simulink model "BL_CollectivePitch_Shutdown"  (R2018a)
settings: Solver=FixedStepAuto  StartTime=0.0  StopTime=FA.TMax  RelTol=1e-3
values from neighbouring files (symbols this model uses):
  FaultDelay = 1    [B_DLC_1_1.m]    (also in B_DLC_1_3.m; B_DLC_1_4.m; B_DLC_1_5.m; B_DLC_2_2.m)
  GenTorqueStopRate = 800/1e3    (= 0.8)    [B_DLC_1_1.m]    (also in B_DLC_1_3.m; B_DLC_1_4.m; B_DLC_1_5.m; B_DLC_2_2.m)
  PitchFaultTime = FA.TMax + 100    [B_DLC_1_1.m]    (also in B_DLC_1_3.m; B_DLC_1_4.m; B_DLC_1_5.m; B_DLC_2_2.m = PitchFaultTimeArray(iFaultTime))
  PitchRampRate1 = 12    [B_DLC_1_1.m]    (also in B_DLC_1_3.m; B_DLC_1_4.m; B_DLC_1_5.m; B_DLC_2_2.m)
  PitchRampRate2 = 2    [B_DLC_1_1.m]    (also in B_DLC_1_3.m; B_DLC_1_4.m; B_DLC_1_5.m; B_DLC_2_2.m)
  PitchRunawayRate = 18    [B_DLC_1_1.m]    (also in B_DLC_1_3.m; B_DLC_1_4.m; B_DLC_1_5.m; B_DLC_2_2.m)
  runawayBlade = 0    [B_DLC_1_1.m]    (also in B_DLC_1_3.m; B_DLC_1_4.m; B_DLC_1_5.m; B_DLC_2_2.m)
  stuckBlade = 0    [B_DLC_1_1.m]    (also in B_DLC_1_3.m; B_DLC_1_4.m; B_DLC_1_5.m; B_DLC_2_2.m)
  YawPzn = Yaw(iYaw)*pi/180    [B_DLC_6_1.m]
  YawRate = 0    [B_DLC_6_1.m]
undefined symbols (not defined in the file or in its folder): Control, DiscIntNeverNeededParam, OLControlParams, OutList, Parameters, PitchControlParams, rpm2radps, S_ConstTq, S_LowBPLim, strmatch, TorqueControlParams
libraries: simulink_extras x1
settings Model: ExtModeTrigMode=oneshot  ExtModeArmWhenConnect=off  Creator=Hazim Namik  LastModifiedBy=dmartin
settings DataIOCC: LimitDataPoints=on  SaveFormat=Array  SignalLoggingName=sigsOut
settings OptimizationCC: BlockReduction=off  BooleanDataType=off  LifeSpan=inf
settings DebuggingCC: SaveWithParameterizedLinksMsg=none  UnderspecifiedInitializationDetection=Classic  MergeDetectMultiDrivingBlocksExec=none  SignalResolutionControl=TryResolveAllWithWarning  AllowSymbolicDim=off  SFUnexpectedBacktrackingDiag=warning  SFNoUnconditionalDefaultTransitionDiag=warning  SFExecutionAtInitializationDiag=none
settings HardwareCC: ProdBitPerPointer=32  ProdBitPerSizeT=32  ProdBitPerPtrDiffT=32  ProdLargestAtomicFloat=None  ProdIntDivRoundTo=Undefined  ProdEndianess=Unspecified  ProdWordSize=32  ProdHWDeviceType=32-bit Generic  TargetBitPerPointer=64  TargetBitPerSizeT=64  TargetBitPerPtrDiffT=64  TargetLongLongMode=on  TargetIntDivRoundTo=Zero  TargetEndianess=LittleEndian  TargetWordSize=64  TargetHWDeviceType=MATLAB Host  ProdEqTarget=off
settings ModelReferenceCC: PropagateSignalLabelsOutOfModel=off
settings CodeAppCC: StateflowObjectComments=on
settings GRTTargetCC: TargetLangStandard=C89/C90 (ANSI)  GeneratePreprocessorConditionals=Disable all
settings ConfigComp: CovMetricSettings=dw  CovHtmlReporting=on  CovSaveCumulativeToWorkspaceVar=on  CovSaveSingleToWorkspaceVar=on  CovExternalEMLEnable=off  CovSFcnEnable=off

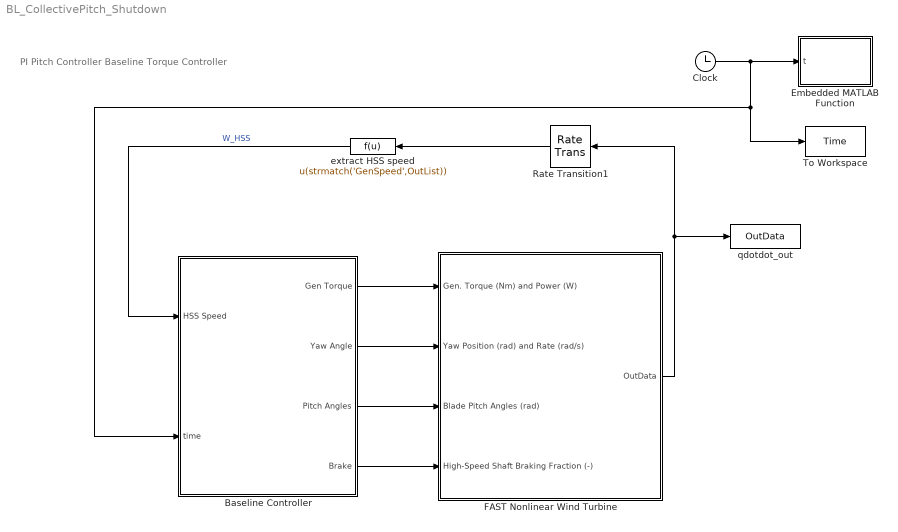
== system BL_CollectivePitch_Shutdown ==
  note: PI Pitch Controller
      | Baseline Torque Controller
  Baseline Controller : Subsystem
  Clock : Clock
  Embedded MATLAB Function : MATLAB Function  TreatAsAtomicUnit=on
  FAST Nonlinear Wind Turbine : Subsystem  mask(FAST Nonlinear Wind Turbine){}
      mask help: This block contains the FAST S-Function.
      mask init:
      | clear FAST_SFunc
  Rate Transition1 : RateTransition
  To Workspace : ToWorkspace  VariableName=Time  SampleTime=-1
  extract HSS speed : Fcn  Expr=u(strmatch('GenSpeed',OutList))
  qdotdot_out : ToWorkspace  VariableName=OutData  SaveFormat=Structure With Time  SampleTime=-1
  wires:
  FAST Nonlinear Wind Turbine/1(OutData) -> Rate Transition1/1, qdotdot_out/1
  Clock/1 -> Baseline Controller/2(time), To Workspace/1, Embedded MATLAB Function/1(t)
  extract HSS speed/1 -> Baseline Controller/1(HSS Speed)  "W_HSS"
  Baseline Controller/1(Gen Torque) -> FAST Nonlinear Wind Turbine/1(Gen. Torque (Nm) and Power (W))
  Baseline Controller/2(Yaw Angle) -> FAST Nonlinear Wind Turbine/2(Yaw Position (rad) and Rate (rad/s))
  Baseline Controller/3(Pitch Angles) -> FAST Nonlinear Wind Turbine/3(Blade Pitch Angles (rad))
  Baseline Controller/4(Brake) -> FAST Nonlinear Wind Turbine/4(High-Speed Shaft Braking Fraction (-))
  Rate Transition1/1 -> extract HSS speed/1

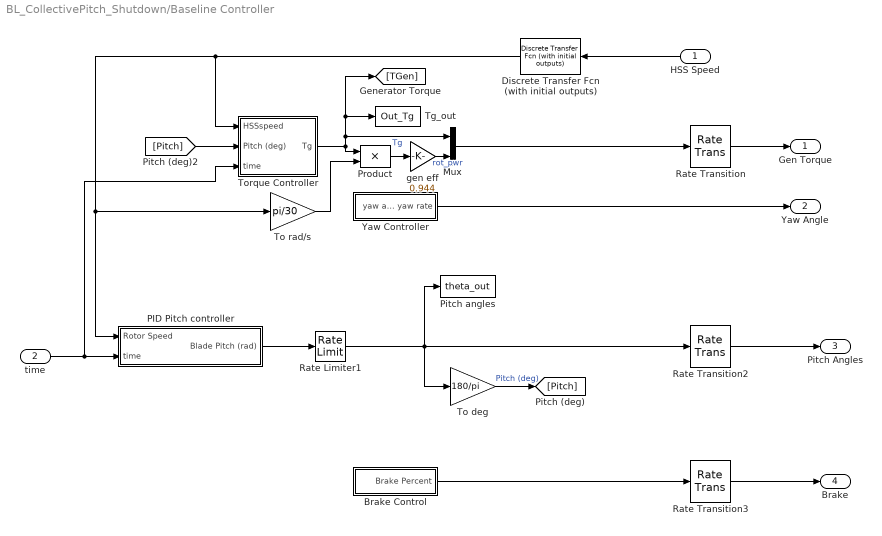
== system BL_CollectivePitch_Shutdown/Baseline Controller ==
  HSS Speed : Inport
  time : Inport  Port=2
  Brake Control : Subsystem
  Discrete Transfer Fcn (with initial outputs) : simulink_extras/Additional Discrete/Discrete Transfer Fcn (with initial outputs)  N=Parameters.LPF.LPnum  D=Parameters.LPF.LPden  U0=Parameters.Turbine.IC.Wr*Parameters.Turbine.G  Y0=Parameters.Turbine.IC.Wr*Parameters.Turbine.G  TS=Control.DT
      settings: SourceProductName=Simulink  SourceProductBaseCode=SL
  Mux : Mux  Inputs=2
  PID Pitch controller : Subsystem
      settings: MinAlgLoopOccurrences=on
  "Pitch angles " : ToWorkspace  VariableName=theta_out  SampleTime=-1
  Product : Product  RndMeth=Zero
  Rate Limiter1 : RateLimiter  RisingSlewLimit=Parameters.PitchActuator.Rate*pi/180  FallingSlewLimit=-Parameters.PitchActuator.Rate*pi/180  SampleTimeMode=inherited  InitialCondition=deg2rad(0)
  Rate Transition : RateTransition  InitialCondition=[0,0]
  Rate Transition2 : RateTransition  InitialCondition=deg2rad(0)
  Rate Transition3 : RateTransition
  Tg_out : ToWorkspace  VariableName=Out_Tg  SampleTime=-1
      settings: MaxDataPoints=Inf
  To deg : Gain  Gain=180/pi
  To rad/s : Gain  Gain=pi/30
  Torque Controller : Subsystem
  Yaw Controller : Subsystem
  gen eff : Gain  Gain=0.944
  Gen Torque : Outport
  Yaw Angle : Outport  Port=2
  Pitch Angles : Outport  Port=3
  Brake : Outport  Port=4
  wires:
  Mux/1 -> Rate Transition/1
  To deg/1 -> [Pitch]  "Pitch (deg)"
  Product/1 -> gen eff/1
  gen eff/1 -> Mux/2  "rot_pwr"
  Discrete Transfer Fcn (with initial outputs)/1 -> Torque Controller/1(HSSspeed), To rad/s/1, PID Pitch controller/1(Rotor Speed)
  [Pitch] -> Torque Controller/2(Pitch (deg))
  Torque Controller/1(Tg) -> Tg_out/1, [TGen], Mux/1, Product/1  "Tg"
  To rad/s/1 -> Product/2
  HSS Speed/1 -> Discrete Transfer Fcn (with initial outputs)/1
  Brake Control/1(Brake Percent) -> Rate Transition3/1
  Rate Transition/1 -> Gen Torque/1
  Yaw Controller/1(yaw and yaw rate) -> Yaw Angle/1
  Rate Transition3/1 -> Brake/1
  PID Pitch controller/1(Blade Pitch (rad)) -> Rate Limiter1/1
  time/1 -> Torque Controller/3(time), PID Pitch controller/2(time)
  Rate Transition2/1 -> Pitch Angles/1
  Rate Limiter1/1 -> "Pitch angles "/1, Rate Transition2/1, To deg/1

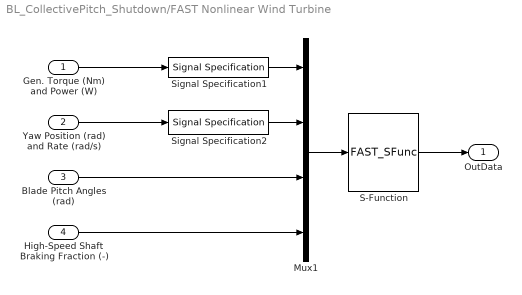
== system BL_CollectivePitch_Shutdown/FAST Nonlinear Wind Turbine ==
  Gen. Torque (Nm) and Power (W) : Inport
  Yaw Position (rad) and Rate (rad/s) : Inport  Port=2
  Blade Pitch Angles (rad) : Inport  Port=3
  High-Speed Shaft Braking Fraction (-) : Inport  Port=4
  Mux1 : Mux
  S-Function : S-Function  FunctionName=FAST_SFunc  Parameters=FAST_InputFileName, FA.TMax, 0  SFunctionDeploymentMode=off  EnableBusSupport=off
  Signal Specification1 : SignalSpecification  OutDataTypeStr=double  Dimensions=2
  Signal Specification2 : SignalSpecification  OutDataTypeStr=double  Dimensions=2
  OutData : Outport
  wires:
  Gen. Torque (Nm) and Power (W)/1 -> Signal Specification1/1
  S-Function/1 -> OutData/1
  Mux1/1 -> S-Function/1
  Blade Pitch Angles (rad)/1 -> Mux1/3
  Yaw Position (rad) and Rate (rad/s)/1 -> Signal Specification2/1
  Signal Specification1/1 -> Mux1/1
  Signal Specification2/1 -> Mux1/2
  High-Speed Shaft Braking Fraction (-)/1 -> Mux1/4

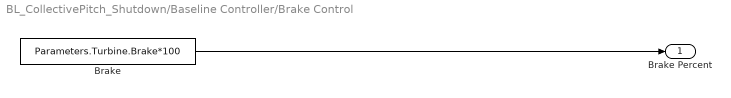
== system BL_CollectivePitch_Shutdown/Baseline Controller/Brake Control ==
  Brake : Constant  Value=Parameters.Turbine.Brake*100
  Brake Percent : Outport
  wires:
  Brake/1 -> Brake Percent/1

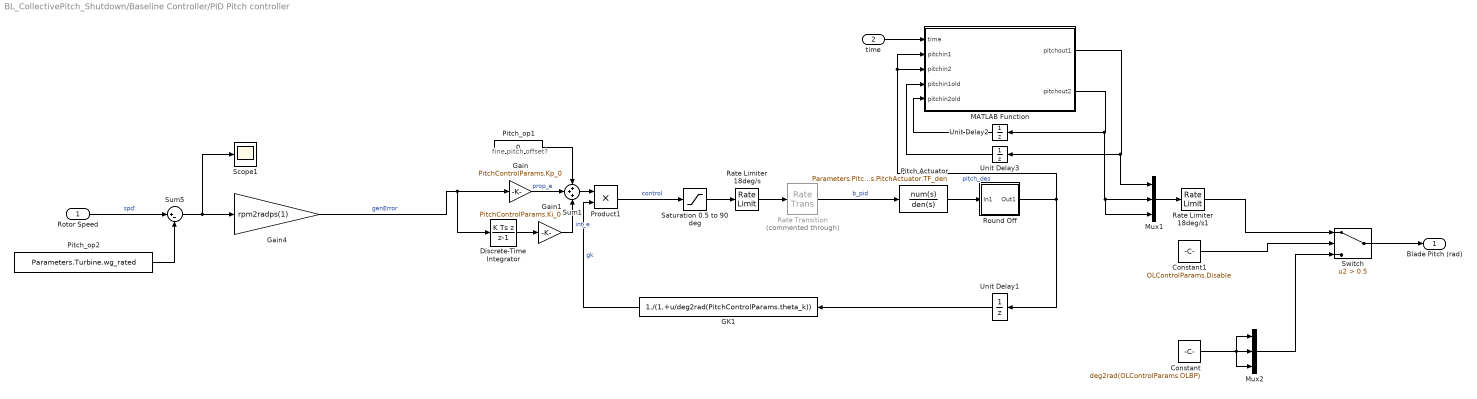
== system BL_CollectivePitch_Shutdown/Baseline Controller/PID Pitch controller ==
  note: fine pitch offset?
  Rotor Speed : Inport
  time : Inport  Port=2
  Constant : Constant  Value=deg2rad(OLControlParams.OLBP)
  Constant1 : Constant  Value=OLControlParams.Disable
  Discrete-Time Integrator : DiscreteIntegrator  IntegratorMethod=Integration: Backward Euler  gainval=1  InitialCondition=deg2rad(Parameters.Turbine.fine_pitch)/(PitchControlParams.Ki_0)/(1./(1.+deg2rad(Parameters.Turbine.fine_pitch)/PitchControlParams.theta_k))  SampleTime=Control.DT  LimitOutput=on  UpperSaturationLimit=5*1.570796/(PitchControlParams.Ki_0)/(1./(1.+1.570796/PitchControlParams.theta_k))  LowerSaturationLimit=deg2rad(Parameters.Turbine.fine_pitch)/(PitchControlParams.Ki_0)/(1./(1.+deg2rad(Parameters.Turbine.fine_pitch)/PitchControlParams.theta_k))  ICPrevOutput=DiscIntNeverNeededParam  ICPrevScaledInput=DiscIntNeverNeededParam
  GK1 : Fcn  Expr=1./(1.+u/deg2rad(PitchControlParams.theta_k))
  Gain : Gain  Gain=PitchControlParams.Kp_0
  Gain1 : Gain  Gain=PitchControlParams.Ki_0
  Gain4 : Gain  Gain=rpm2radps(1)
  MATLAB Function : MATLAB Function  TreatAsAtomicUnit=on
  Mux1 : Mux  Inputs=3
  Mux2 : Mux  Inputs=3
  Pitch Actuator : TransferFcn  Numerator=Parameters.PitchActuator.TF_num  Denominator=Parameters.PitchActuator.TF_den
  Pitch_op1 : Constant  Value=0  SampleTime=Control.DT
  Pitch_op2 : Constant  Value=Parameters.Turbine.wg_rated  SampleTime=Control.DT
  Product1 : Product  RndMeth=Zero
  Rate Limiter 18deg/s : RateLimiter  RisingSlewLimit=Parameters.PitchActuator.Rate*pi/180  FallingSlewLimit=-Parameters.PitchActuator.Rate*pi/180  SampleTimeMode=inherited  InitialCondition=deg2rad(0)
  Rate Limiter 18deg/s1 : RateLimiter  RisingSlewLimit=Parameters.PitchActuator.Rate*pi/180  FallingSlewLimit=-Parameters.PitchActuator.Rate*pi/180  SampleTimeMode=inherited  InitialCondition=deg2rad(0)
  Rate Transition : RateTransition  Commented=through
  Round Off : Subsystem
  Saturation 0.5 to 90 deg : Saturate  UpperLimit=90*pi/180  LowerLimit=deg2rad(Parameters.Turbine.fine_pitch)
  Scope1 : Scope
  Sum1 : Sum  Inputs=+++
  Sum5 : Sum  Inputs=|+-  SaturateOnIntegerOverflow=on  InputSameDT=on  OutDataTypeStr=Inherit: Same as first input
  Switch : Switch  Criteria=u2 > Threshold  Threshold=0.5
  Unit Delay1 : UnitDelay  InitialCondition=Parameters.Turbine.IC.Bp  SampleTime=Control.DT
  Unit Delay2 : UnitDelay  InitialCondition=Parameters.Turbine.IC.Bp  SampleTime=Control.DT
  Unit Delay3 : UnitDelay  InitialCondition=Parameters.Turbine.IC.Bp  SampleTime=Control.DT
  Blade Pitch (rad) : Outport
  wires:
  Pitch_op2/1 -> Sum5/2
  Rotor Speed/1 -> Sum5/1  "spd'"
  Discrete-Time Integrator/1 -> Gain1/1
  Gain/1 -> Sum1/2  "prop_e"
  Pitch_op1/1 -> Sum1/1
  Gain1/1 -> Sum1/3  "int_e"
  Sum1/1 -> Product1/1
  Unit Delay1/1 -> GK1/1
  Saturation 0.5 to 90 deg/1 -> Rate Limiter 18deg/s/1
  GK1/1 -> Product1/2  "gk"
  Rate Transition/1 -> Pitch Actuator/1  "b_pid"
  Rate Limiter 18deg/s/1 -> Rate Transition/1
  Sum5/1 -> Scope1/1, Gain4/1
  Product1/1 -> Saturation 0.5 to 90 deg/1  "control"
  Gain4/1 -> Discrete-Time Integrator/1, Gain/1  "genError"
  Mux1/1 -> Rate Limiter 18deg/s1/1
  Switch/1 -> Blade Pitch (rad)/1
  Constant1/1 -> Switch/2
  Constant/1 -> Mux2/1, Mux2/3, Mux2/2
  Mux2/1 -> Switch/3
  Pitch Actuator/1 -> Round Off/1(In1)
  time/1 -> MATLAB Function/1(time)
  MATLAB Function/1(pitchout1) -> Mux1/1, Unit Delay3/1
  MATLAB Function/2(pitchout2) -> Mux1/3, Mux1/2, Unit Delay2/1
  Unit Delay2/1 -> MATLAB Function/5(pitchin2old)
  Unit Delay3/1 -> MATLAB Function/4(pitchin1old)
  Round Off/1(Out1) -> MATLAB Function/3(pitchin2), MATLAB Function/2(pitchin1), Unit Delay1/1  "pitch_des"
  Rate Limiter 18deg/s1/1 -> Switch/1

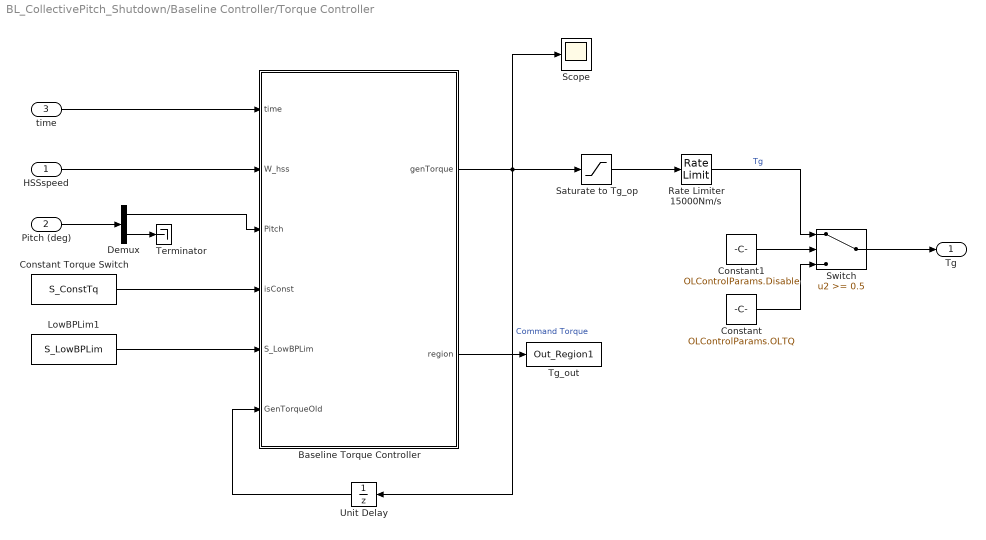
== system BL_CollectivePitch_Shutdown/Baseline Controller/Torque Controller ==
  HSSspeed : Inport
  Pitch (deg) : Inport  Port=2
  time : Inport  Port=3
  Baseline Torque Controller : MATLAB Function  TreatAsAtomicUnit=on
  Constant : Constant  Value=OLControlParams.OLTQ
  Constant Torque Switch : Constant  Value=S_ConstTq  SampleTime=Control.DT
  Constant1 : Constant  Value=OLControlParams.Disable
  Demux : Demux  Outputs=[1, 2]
  LowBPLim1 : Constant  Value=S_LowBPLim  SampleTime=Control.DT
  Rate Limiter 15000Nm/s : RateLimiter  RisingSlewLimit=15000  FallingSlewLimit=-15000  SampleTimeMode=inherited
  Saturate to Tg_op : Saturate  UpperLimit=TorqueControlParams.T_rated  LowerLimit=0
  Scope : Scope
  Switch : Switch  Threshold=0.5
  Terminator : Terminator
  Tg_out : ToWorkspace  VariableName=Out_Region1  SampleTime=-1
      settings: MaxDataPoints=Inf
  Unit Delay : UnitDelay  InitialCondition=Parameters.Turbine.IC.Tg  SampleTime=-1
  Tg : Outport
  wires:
  Pitch (deg)/1 -> Demux/1
  Demux/2 -> Terminator/1
  Saturate to Tg_op/1 -> Rate Limiter 15000Nm/s/1
  Switch/1 -> Tg/1
  Constant/1 -> Switch/3
  Rate Limiter 15000Nm/s/1 -> Switch/1  "Tg"
  Constant1/1 -> Switch/2
  Baseline Torque Controller/1(genTorque) -> Unit Delay/1, Saturate to Tg_op/1, Scope/1  "Command Torque"
  Baseline Torque Controller/2(region) -> Tg_out/1
  HSSspeed/1 -> Baseline Torque Controller/2(W_hss)
  Constant Torque Switch/1 -> Baseline Torque Controller/4(isConst)
  LowBPLim1/1 -> Baseline Torque Controller/5(S_LowBPLim)
  Demux/1 -> Baseline Torque Controller/3(Pitch)
  time/1 -> Baseline Torque Controller/1(time)
  Unit Delay/1 -> Baseline Torque Controller/6(GenTorqueOld)

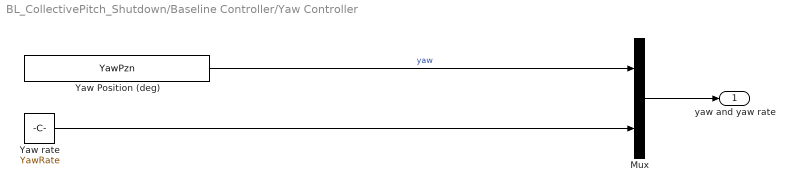
== system BL_CollectivePitch_Shutdown/Baseline Controller/Yaw Controller ==
  Mux : Mux  Inputs=2
  Yaw Position (deg) : Constant  Value=YawPzn  SampleTime=-1
  Yaw rate : Constant  Value=YawRate  SampleTime=-1
  yaw and yaw rate : Outport
  wires:
  Mux/1 -> yaw and yaw rate/1
  Yaw Position (deg)/1 -> Mux/1  "yaw"
  Yaw rate/1 -> Mux/2

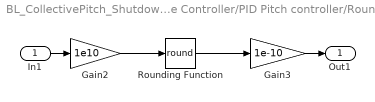
== system BL_CollectivePitch_Shutdown/Baseline Controller/PID Pitch controller/Round Off ==
  In1 : Inport
  Gain2 : Gain  Gain=1e10
  Gain3 : Gain  Gain=1e-10
  Rounding Function : Rounding  Operator=round
  Out1 : Outport
  wires:
  Gain2/1 -> Rounding Function/1
  Rounding Function/1 -> Gain3/1
  Gain3/1 -> Out1/1
  In1/1 -> Gain2/1

== matlab function BL_CollectivePitch_Shutdown/Baseline Controller/PID Pitch controller/MATLAB Function ==
  data: time input; pitchout1 output; pitchout2 output; pitchin1 input; pitchin2 input; pitchin1old input; pitchin2old input; PitchFaultTime parameter; PitchRampRate1 parameter; PitchRampRate2 parameter; FaultDelay parameter; Control parameter; PitchRunawayRate parameter; stuckBlade parameter; runawayBlade parameter
function [pitchout1,pitchout2] = fcn(time,pitchin1,pitchin2,pitchin1old,pitchin2old,PitchFaultTime,PitchRampRate1,PitchRampRate2,FaultDelay,Control,PitchRunawayRate, stuckBlade, runawayBlade)

if stuckBlade == 1
    if time >= PitchFaultTime && time < PitchFaultTime + FaultDelay
        pitchout1 = pitchin1old; % blade1 is stuck
        pitchout2 = pitchin2;
    elseif time >= PitchFaultTime + FaultDelay && pitchin2old < 90*pi/180 && time < PitchFaultTime + FaultDelay + 3
        pitchout1 = pitchin1old; % blade1 is stuck
        pitchout2 = PitchRampRate1*pi/180*Control.DT + pitchin2old; % pitch at 18 deg/s (time-step of 0.0125s)
        if pitchout2 > 90*pi/180
            pitchout2 = 90*pi/180;
        end
    elseif time >= PitchFaultTime + FaultDelay + 3 && pitchin2old < 90*pi/180
        pitchout1 = pitchin1old; % blade1 is stuck
        pitchout2 = PitchRampRate2*pi/180*Control.DT + pitchin2old; % pitch at 2 deg/s (time-step of 0.0125s)
        if pitchout2 > 90*pi/180
            pitchout2 = 90*pi/180;
        end
    elseif time >= PitchFaultTime + FaultDelay && pitchin2old >= 90*pi/180
        pitchout1 = pitchin1old; % blade1 is stuck
        pitchout2 = 90*pi/180; % blade2 is feathered
    else
        pitchout1 = pitchin1; % normal operation
        pitchout2 = pitchin2; % normal operation
    end
elseif runawayBlade == 1
    if time >= PitchFaultTime && time < PitchFaultTime + FaultDelay
        pitchout1 = -PitchRunawayRate*pi/180*Control.DT + pitchin1old; % blade1 is running away
        pitchout2 = pitchin2;
        if pitchout1 < -10*pi/180
            pitchout1 = -10*pi/180;
        end
    elseif time >= PitchFaultTime + FaultDelay && pitchin2old < 90*pi/180 && time < PitchFaultTime + FaultDelay + 3
        pitchout1 = -PitchRunawayRate*pi/180*Control.DT + pitchin1old; % blade1 is running away
        pitchout2 = PitchRampRate1*pi/180*Control.DT + pitchin2old; % pitch at 18 deg/s (time-step of 0.0125s)
        if pitchout1 < -10*pi/180
            pitchout1 = -10*pi/180;
        end
        if pitchout2 > 90*pi/180
            pitchout2 = 90*pi/180;
        end
    elseif time >= PitchFaultTime + FaultDelay && pitchin2old < 90*pi/180
        pitchout1 = -PitchRunawayRate*pi/180*Control.DT + pitchin1old; % blade1 is running away
        pitchout2 = PitchRampRate2*pi/180*Control.DT + pitchin2old; % pitch at 18 deg/s (time-step of 0.0125s)
        if pitchout1 < -10*pi/180
            pitchout1 = -10*pi/180;
        end
        if pitchout2 > 90*pi/180
            pitchout2 = 90*pi/180;
        end
    elseif time >= PitchFaultTime + FaultDelay && pitchin2old >= 90*pi/180
        pitchout1 = -PitchRunawayRate*pi/180*Control.DT + pitchin1old; % blade1 is running away
        pitchout2 = 90*pi/180; % blade2 is feathered
        if pitchout1 < -10*pi/180
            pitchout1 = -10*pi/180;
        end
    else
        pitchout1 = pitchin1; % normal operation
        pitchout2 = pitchin2; % normal operation
    end
else
    pitchout1 = pitchin1; % normal operation
    pitchout2 = pitchin2; % normal operation
end

== matlab function BL_CollectivePitch_Shutdown/Embedded MATLAB Function ==
  data: t input
function TellTime(t)

if t==0
    Tsim=t
elseif rem(t,50)==0
    Tsim=t
end

== matlab function BL_CollectivePitch_Shutdown/Baseline Controller/Torque Controller/Baseline Torque Controller ==
  settings: updateMethod=DISCRETE  sampleTime=Control.DT
  data: time input; W_hss input; Pitch input; genTorque output; isConst input; region output; S_LowBPLim input; GenTorqueOld input; TorqueControlParams parameter; PitchFaultTime parameter; Control parameter; GenTorqueStopRate parameter
function [genTorque, region] = regionSelectTq_Flex( time, W_hss, Pitch, isConst, S_LowBPLim, GenTorqueOld, TorqueControlParams, PitchFaultTime, Control, GenTorqueStopRate)
% This block supports an embeddable subset of the MATLAB language.
% See the help menu for details.


%% Assign Constants

wg_rated    = TorqueControlParams.wg_rated;
T_rated     = TorqueControlParams.T_rated;
w2_high     = TorqueControlParams.w2_high;
w1_high     = TorqueControlParams.w1_high;
wg_min      = TorqueControlParams.wg_min;
m2_5        = TorqueControlParams.m2_5;
c2_5        = TorqueControlParams.c2_5;
m1_5        = TorqueControlParams.m1_5;
c1_5        = TorqueControlParams.c1_5;
k_opt       = TorqueControlParams.k_opt;
P0          = TorqueControlParams.P0;
T2_high     = m2_5 * w2_high + c2_5;

%% Switch based on Gen. Speed

if time >= PitchFaultTime
    genTorque = GenTorqueOld - GenTorqueOld*GenTorqueStopRate*Control.DT;
    region = 4;
    if genTorque < 0
        genTorque = 0;
    end    
elseif (((S_LowBPLim==0)&&(W_hss >= wg_rated)) || ((S_LowBPLim==1)&&((Pitch >= TorqueControlParams.fine_pitch+3) || (W_hss >= wg_rated)))) %Region 3 calcs
    region=3;
    if (isConst)
        genTorque = T_rated;
    else
        genTorque = 30/pi * P0 / W_hss;
    end
elseif (W_hss >= w2_high)                %Region 2.5
    region=2.5;    
    genTorque = m2_5 * W_hss + c2_5;
    
elseif (W_hss >= w1_high)                    %Region 2
    region=2;
    genTorque = k_opt * W_hss^2;
elseif (W_hss > wg_min)                    %Region 1.5
    region=1.5;
    genTorque = m1_5 * W_hss + c1_5;
else                                    %Region 1
    region=1;
    genTorque = 0;
end
